simulink model "Ejercicio15"  (R2012b)
settings: Solver=ode45  StartTime=0.0  StopTime=10.0  RelTol=1e-3
values from neighbouring files (symbols this model uses):
  a = [0 1 0 0; 20.601 0 0 0; 0 0 0 1; -0.4905 0 0 0]    [ejercicio15.m]
  b = [0; -1 ; 0;0.5]    [ejercicio15.m]
  c = [0 0 1 0]    [ejercicio15.m]
  h = h'    [ejercicio15.m]
  k = acker(a,b,pd)    [ejercicio15.m]
  ki = kt(1,5)    [ejercicio15.m]
  kp = kt(1,1:4)    [ejercicio15.m]
settings Model: Creator=mario  LastModifiedBy=carlos_mar.paredes
settings DataIOCC: SignalLoggingSaveFormat=ModelDataLogs
settings OptimizationCC: ExpressionDepthLimit=128
settings DebuggingCC: MultiTaskDSMMsg=warning  MultiTaskCondExecSysMsg=none  StrictBusMsg=None
settings RTWCC: IncludeERTFirstTime=on
settings CodeAppCC: CustomSymbolStrType=$N$R$M_T  InternalIdentifier=Shortened

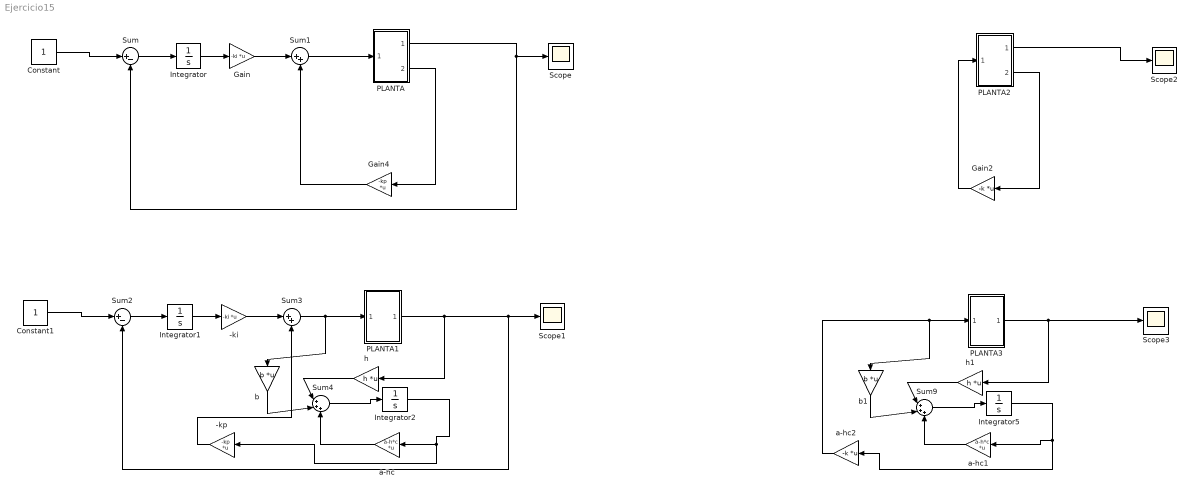
== system Ejercicio15 ==
  "-ki " : Gain  Gain=-ki  Multiplication=Matrix(K*u) (u vector)
  -kp : Gain  Gain=-kp  Multiplication=Matrix(K*u) (u vector)
  Constant : Constant
  Constant1 : Constant
  Gain : Gain  Gain=-ki  Multiplication=Matrix(K*u) (u vector)
  Gain2 : Gain  Gain=-k  Multiplication=Matrix(K*u) (u vector)
  Gain4 : Gain  Gain=-kp  Multiplication=Matrix(K*u) (u vector)
  Integrator : Integrator
  Integrator1 : Integrator
  Integrator2 : Integrator
  Integrator5 : Integrator  InitialCondition=[1 1 1 1]
  PLANTA : Subsystem
  PLANTA1 : Subsystem
  PLANTA2 : Subsystem
  PLANTA3 : Subsystem
  Scope{,1..3} (4 alike) : Scope
      Scope2 settings: SaveName=ScopeData2
      Scope3 settings: SaveName=ScopeData3
  Sum : Sum  Inputs=|+-
  Sum1 : Sum  Inputs=|++
  Sum2 : Sum  Inputs=|+-
  Sum3 : Sum  Inputs=|++
  Sum4 : Sum  Inputs=|+++
  Sum9 : Sum  Inputs=|+++
  a-hc : Gain  Gain=a-h*c  Multiplication=Matrix(K*u) (u vector)
  a-hc1 : Gain  Gain=a-h*c  Multiplication=Matrix(K*u) (u vector)
  a-hc2 : Gain  Gain=-k  Multiplication=Matrix(K*u) (u vector)
  b : Gain  Gain=b  Multiplication=Matrix(K*u) (u vector)
  b1 : Gain  Gain=b  Multiplication=Matrix(K*u) (u vector)
  h : Gain  Gain=h  Multiplication=Matrix(K*u) (u vector)
  h1 : Gain  Gain=h  Multiplication=Matrix(K*u) (u vector)
  wires:
  Sum/1 -> Integrator/1
  Integrator/1 -> Gain/1
  Gain/1 -> Sum1/1
  Gain4/1 -> Sum1/2
  Constant/1 -> Sum/1
  PLANTA/1(Out1) -> Sum/2, Scope/1
  Sum1/1 -> PLANTA/1(In1)
  PLANTA/2(Out2) -> Gain4/1
  Sum2/1 -> Integrator1/1
  Integrator1/1 -> "-ki "/1
  "-ki "/1 -> Sum3/1
  Constant1/1 -> Sum2/1
  PLANTA1/1(Out1) -> h/1, Scope1/1, Sum2/2
  Sum3/1 -> b/1, PLANTA1/1(In1)
  h/1 -> Sum4/1
  b/1 -> Sum4/2
  Sum4/1 -> Integrator2/1
  Integrator2/1 -> -kp/1, a-hc/1
  a-hc/1 -> Sum4/3
  -kp/1 -> Sum3/2
  PLANTA2/1(Out1) -> Scope2/1
  Gain2/1 -> PLANTA2/1(In1)
  PLANTA2/2(Out2) -> Gain2/1
  PLANTA3/1(Out1) -> h1/1, Scope3/1
  a-hc2/1 -> b1/1, PLANTA3/1(In1)
  h1/1 -> Sum9/1
  b1/1 -> Sum9/2
  Sum9/1 -> Integrator5/1
  Integrator5/1 -> a-hc2/1, a-hc1/1
  a-hc1/1 -> Sum9/3

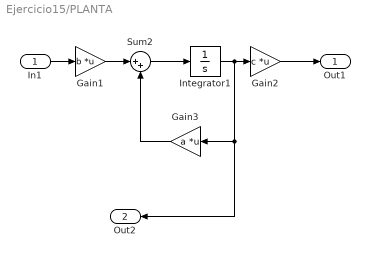
== system Ejercicio15/PLANTA ==
  In1 : Inport
  Gain1 : Gain  Gain=b  Multiplication=Matrix(K*u) (u vector)
  Gain2 : Gain  Gain=c  Multiplication=Matrix(K*u) (u vector)
  Gain3 : Gain  Gain=a  Multiplication=Matrix(K*u) (u vector)
  Integrator1 : Integrator
  Sum2 : Sum  Inputs=|++
  Out1 : Outport
  Out2 : Outport  Port=2
  wires:
  Integrator1/1 -> Out2/1, Gain3/1, Gain2/1
  In1/1 -> Gain1/1
  Gain1/1 -> Sum2/1
  Gain3/1 -> Sum2/2
  Gain2/1 -> Out1/1
  Sum2/1 -> Integrator1/1

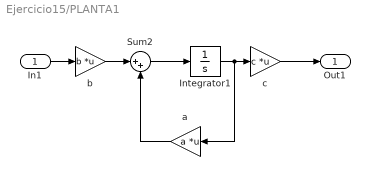
== system Ejercicio15/PLANTA1 ==
  In1 : Inport
  Integrator1 : Integrator
  Sum2 : Sum  Inputs=|++
  a : Gain  Gain=a  Multiplication=Matrix(K*u) (u vector)
  b : Gain  Gain=b  Multiplication=Matrix(K*u) (u vector)
  c : Gain  Gain=c  Multiplication=Matrix(K*u) (u vector)
  Out1 : Outport
  wires:
  Sum2/1 -> Integrator1/1
  c/1 -> Out1/1
  a/1 -> Sum2/2
  b/1 -> Sum2/1
  In1/1 -> b/1
  Integrator1/1 -> c/1, a/1

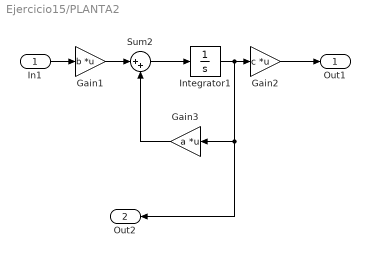
== system Ejercicio15/PLANTA2 ==
  In1 : Inport
  Gain1 : Gain  Gain=b  Multiplication=Matrix(K*u) (u vector)
  Gain2 : Gain  Gain=c  Multiplication=Matrix(K*u) (u vector)
  Gain3 : Gain  Gain=a  Multiplication=Matrix(K*u) (u vector)
  Integrator1 : Integrator  InitialCondition=[1 1 1 1]
  Sum2 : Sum  Inputs=|++
  Out1 : Outport
  Out2 : Outport  Port=2
  wires:
  Integrator1/1 -> Out2/1, Gain3/1, Gain2/1
  In1/1 -> Gain1/1
  Gain1/1 -> Sum2/1
  Gain3/1 -> Sum2/2
  Gain2/1 -> Out1/1
  Sum2/1 -> Integrator1/1

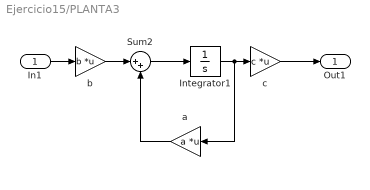
== system Ejercicio15/PLANTA3 ==
  In1 : Inport
  Integrator1 : Integrator  InitialCondition=[1 1 1 1]
  Sum2 : Sum  Inputs=|++
  a : Gain  Gain=a  Multiplication=Matrix(K*u) (u vector)
  b : Gain  Gain=b  Multiplication=Matrix(K*u) (u vector)
  c : Gain  Gain=c  Multiplication=Matrix(K*u) (u vector)
  Out1 : Outport
  wires:
  Sum2/1 -> Integrator1/1
  c/1 -> Out1/1
  a/1 -> Sum2/2
  b/1 -> Sum2/1
  In1/1 -> b/1
  Integrator1/1 -> c/1, a/1
